simulink model "vehicle_test"  (R2018a)
settings: Solver=VariableStepAuto  StartTime=0.0  StopTime=10.0  RelTol=1e-3
undefined symbols (not defined in the file): theta_0, x_0
settings Model: Creator=hkedw  LastModifiedBy=hkedw

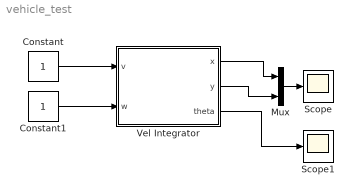
== system vehicle_test ==
  Constant : Constant
  Constant1 : Constant
  Mux : Mux  Inputs=2
  Scope : Scope
  Scope1 : Scope
  Vel Integrator : Subsystem
  wires:
  Constant/1 -> Vel Integrator/1(v)
  Constant1/1 -> Vel Integrator/2(w)
  Vel Integrator/1(x) -> Mux/1
  Vel Integrator/2(y) -> Mux/2
  Vel Integrator/3(theta) -> Scope1/1
  Mux/1 -> Scope/1

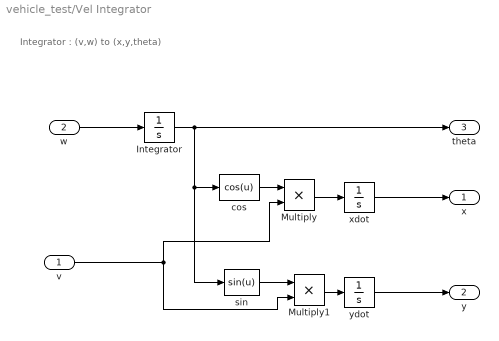
== system vehicle_test/Vel Integrator ==
  note: Integrator : (v,w) to (x,y,theta)
  v : Inport
  w : Inport  Port=2
  Integrator : Integrator  InitialCondition=theta_0
  Multiply : Product
  Multiply1 : Product
  cos : MATLABFcn  MATLABFcn=cos(u)
  sin : MATLABFcn  MATLABFcn=sin(u)
  xdot : Integrator  InitialCondition=x_0
  ydot : Integrator  InitialCondition=x_0
  x : Outport
  y : Outport  Port=2
  theta : Outport  Port=3
  wires:
  w/1 -> Integrator/1
  Multiply/1 -> xdot/1
  cos/1 -> Multiply/1
  Multiply1/1 -> ydot/1
  ydot/1 -> y/1
  xdot/1 -> x/1
  sin/1 -> Multiply1/1
  Integrator/1 -> theta/1, sin/1, cos/1
  v/1 -> Multiply/2, Multiply1/2
